simulink model "FM_PM_modulation"  (R2024a)
settings: Solver=VariableStepAuto  StartTime=0.0  StopTime=10.0  MaxStep=0.001  RelTol=1e-3
libraries: commanapbnd3 x1
settings Model: Creator=zeyad  LastModifiedBy=zeyad

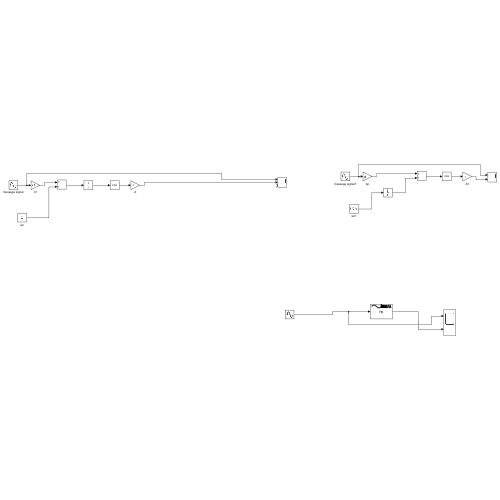
[thumbnail: Simulink's stored preview of the top-level diagram]
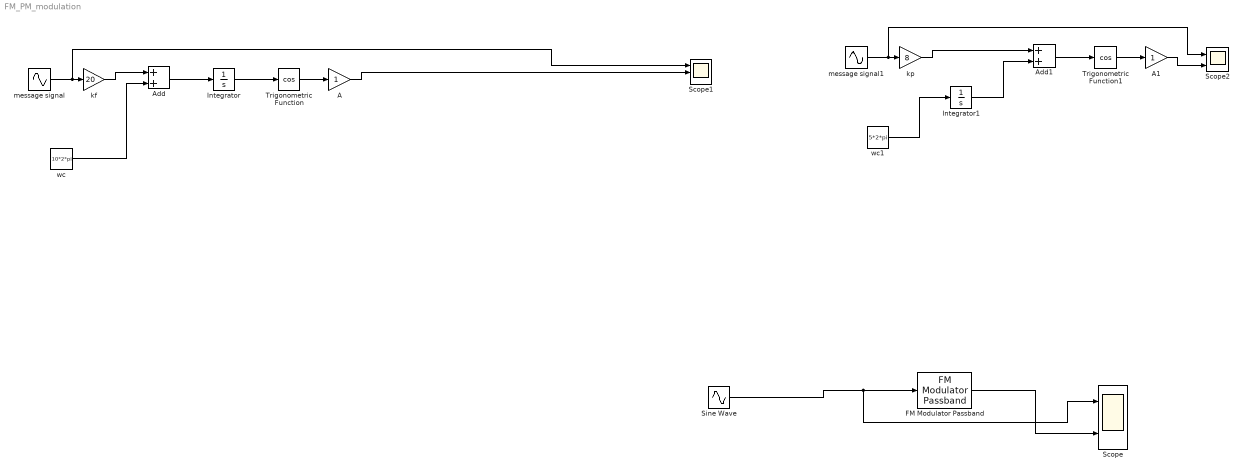
== system FM_PM_modulation ==
  A : Gain
  A1 : Gain
  Add : Sum
  Add1 : Sum
  FM Modulator Passband : commanapbnd3/FM Modulator Passband  Fc=7  Ph=0  Kc=5
  Integrator : Integrator
  Integrator1 : Integrator
  Scope : Scope  NumInputPorts=2
  Scope1 : Scope  NumInputPorts=3
  Scope2 : Scope  NumInputPorts=2
  Sine Wave : Sin  Frequency=2  SampleTime=0.001
  Trigonometric Function : Trigonometry  Operator=cos
  Trigonometric Function1 : Trigonometry  Operator=cos
  kf : Gain  Gain=20
  kp : Gain  Gain=8
  message signal : Sin  Frequency=1*2*pi  SampleTime=0
  message signal1 : Sin  Frequency=1*2*pi  SampleTime=0
  wc : Constant  Value=10*2*pi
  wc1 : Constant  Value=5*2*pi
  wires:
  FM Modulator Passband/1 -> Scope/2
  Sine Wave/1 -> Scope/1, FM Modulator Passband/1
  wc/1 -> Add/2
  kf/1 -> Add/1
  Add/1 -> Integrator/1
  Integrator/1 -> Trigonometric Function/1
  Trigonometric Function/1 -> A/1
  message signal/1 -> Scope1/1, kf/1
  message signal1/1 -> Scope2/1, kp/1
  A1/1 -> Scope2/2
  Trigonometric Function1/1 -> A1/1
  kp/1 -> Add1/1
  Add1/1 -> Trigonometric Function1/1
  wc1/1 -> Integrator1/1
  Integrator1/1 -> Add1/2
  A/1 -> Scope1/2
